simulink model "ADRC_Han"  (R2024b)
settings: Solver=VariableStepAuto  StartTime=0.0  StopTime=20  RelTol=1e-3
values from neighbouring files (symbols this model uses):
  A = [zeros(N, 1)  eye(N, N) ... (first row only)    [ADRC_Han_Vars.m]
  A_d_test = d_test_ss.A    [ADRC_Han_Vars.m]
  A_ESO_d = [1-l1_ESO_d, delta_t-l1_ESO_d*delta_t, 1/2 * delta_t^2 - 1/2 * l1_ESO_d*delta_t^2 ... (first row only)    [ADRC_Han_Vars.m]
  A_MESO_d = A_o_d - l_MESO_d*C_o_d*A_o_d    [ADRC_Han_Vars.m]
  A_o = [A_m e_m*c_T_d_m ... (first row only)    [ADRC_Han_Vars.m]
  A_O_d = A_m_d - l_o_d*C_m_d*A_m_d    [ADRC_Han_Vars.m]
  A_o_lqr = [A_m_lqr e_m*c_T_d_m_lqr ... (first row only)    [ADRC_Han_Vars.m]
  alpha_1 = 1    [ADRC_Han_Vars.m]
  alpha_2 = 1    [ADRC_Han_Vars.m]
  b = [zeros(N-1, 1) ... (first row only)    [ADRC_Han_Vars.m]
  b0 = K/T^2    (= 1.11111111111)    [ADRC_Han_Vars.m]
  B_d_test = d_test_ss.B    [ADRC_Han_Vars.m]
  b_ESO_d = [1/2*b0*delta_t^2 - l1_ESO_d*b0*delta_t^2 ... (first row only)    [ADRC_Han_Vars.m]
  B_MESO_d = B_o_d - l_MESO_d*C_o_d*B_o_d    [ADRC_Han_Vars.m]
  b_o = [b_m ... (first row only)    [ADRC_Han_Vars.m]
  B_O_d = B_m_d - l_o_d*C_m_d*B_m_d    [ADRC_Han_Vars.m]
  b_o_lqr = [b_m_lqr ... (first row only)    [ADRC_Han_Vars.m]
  beta_01 = 1    [ADRC_Han_Vars.m]
  beta_02 = 1 / (2*h^0.5)    (= 5)    [ADRC_Han_Vars.m]
  beta_03 = 2 / (5^2 * h^1.2)    (= 20.0950914521)    [ADRC_Han_Vars.m]
  c = 50    [ADRC_Han_Vars.m]
  C_d_test = d_test_ss.C    [ADRC_Han_Vars.m]
  c_o_T = [c_T_m 0]    [ADRC_Han_Vars.m]
  c_o_T_lqr = [c_T_m_lqr 0]    [ADRC_Han_Vars.m]
  c_t = [1, zeros(1, N)]    [ADRC_Han_Vars.m]
  D = 5    [ADRC_Han_Vars.m]
  delta = 0.05    [ADRC_Han_Vars.m]
  delta_t = 0.01    [ADRC_Han_Vars.m]
  h = 0.01    [ADRC_Han_Vars.m]
  h0 = 8*h    (= 0.08)    [ADRC_Han_Vars.m]
  K = 10    [ADRC_Han_Vars.m]
  k = ones(N,1)    [ADRC_Han_Vars.m]
  k1_c_d = (1 - z_cl)^2/delta_t^2    [ADRC_Han_Vars.m]
  k_c_T = acker(A_m,b_m, [-omega_cl,-omega_cl])    [ADRC_Han_Vars.m]
  k_c_T_dlqr = dlqr(A_m_dlqr,b_m_dlqr,Q,R)    [ADRC_Han_Vars.m]
  k_c_T_lqr = lqr(A_m_lqr,b_m_lqr,Q,R)    [ADRC_Han_Vars.m]
  k_d_T = (e_m*c_T_d_m) \ b_m    [ADRC_Han_Vars.m]
  k_d_T_lqr = (e_m*c_T_d_m_lqr) \ b_m_lqr    [ADRC_Han_Vars.m]
  k_dlqr = dlqr(A_m_d, B_m_d, Q, R)    [ADRC_Han_Vars.m]
  K_lqr = lqr(A_lqr,B_lqr,Q,R)    [ADRC_Han_Vars.m]
  k_o = acker(A_o',c_o_T',[-omega_O,-omega_O,-omega_O])'    [ADRC_Han_Vars.m]
  k_o_lqr = acker(A_o_lqr',c_o_T_lqr',[-omega_O,-omega_O,-omega_O])'    [ADRC_Han_Vars.m]
  k_s = -inv(c_T_m*inv(A_m-b_m*k_c_T)*b_m)    [ADRC_Han_Vars.m]
  k_s_dlqr = -inv(c_T_m*inv(A_m-b_m*k_dlqr)*b_m)    [ADRC_Han_Vars.m]
  k_s_lqr = -inv(c_T_m_lqr*inv(A_m_lqr-b_m_lqr*k_c_T_lqr)*b_m_lqr)    [ADRC_Han_Vars.m]
  K_s_lqr = -inv(C_lqr*inv(A_lqr-B_lqr*K_lqr)*B_lqr)    [ADRC_Han_Vars.m]
  k_T_d = [k1_c_d, k2_c_d]    [ADRC_Han_Vars.m]
  l = ones(N+1, 1)    [ADRC_Han_Vars.m]
  l_ESO_d = [l1_ESO_d, l2_ESO_d, l3_ESO_d]'    [ADRC_Han_Vars.m]
  l_MESO_d = acker(A_o_d',C_o_d',[z_MESO,z_MESO,z_MESO])'    [ADRC_Han_Vars.m]
  l_o_d = acker(A_m_d',C_m_d',[z_o,z_o])'    [ADRC_Han_Vars.m]
  N = 2    [ADRC_Han_Vars.m]
  r = 100000    [ADRC_Han_Vars.m]
  r0 = 2    [ADRC_Han_Vars.m]
  T = 3    [ADRC_Han_Vars.m]
undefined symbols (not defined in the file or in its folder): A_o_dlqr, b_o_dlqr, c_o_T_dlqr
libraries: simulink x2, slpidlib x1
settings Model: Creator=Henrik  LastModifiedBy=Henrik

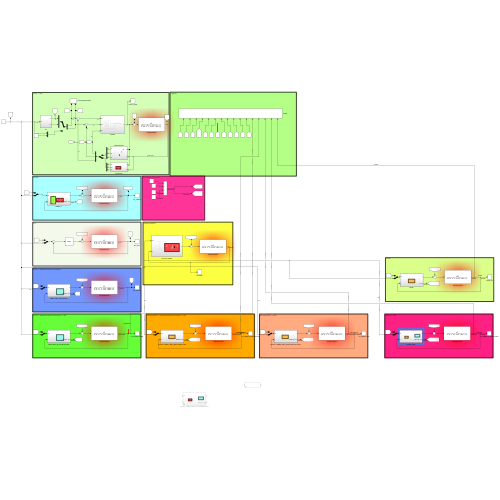
[thumbnail: Simulink's stored preview of the top-level diagram]
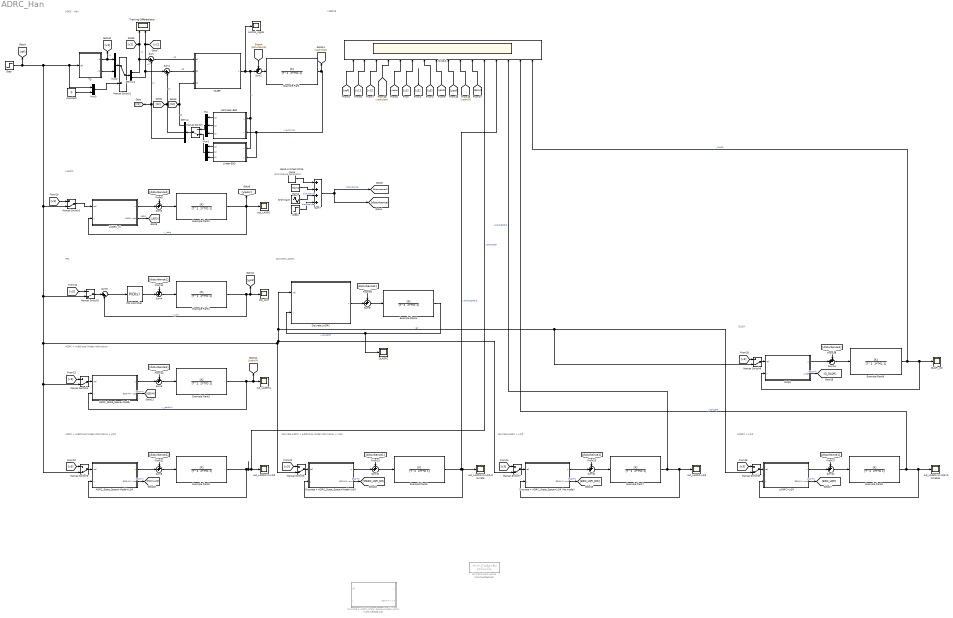
== system ADRC_Han ==
  note: Discrete LADRC
  note: Logging
  note: Disturbance Generation
  note: LADRC
  note: ADRC - Han
  note: PID
  note: ADRC + Additional Model Information
  note: ADRC + Additional Model Information + LQR
  note: Discrete ADRC + Additional Model Information + LQR
  note: Discrete ADRC + LQR
  note: LADRC + LQR
  note: DLQR
   Example Plant{,1..9} (10 alike) : TransferFcn  Numerator=[K]  Denominator="[T^2  2*T*D 1]"
  ADRC_State_Space+Model : Subsystem
  ADRC_State_Space+Model+LQR : Subsystem
  Band-Limited White Noise : simulink/Sources/Band-Limited White Noise  Cov=[0]  Ts=5  seed=[23341]
  Constant : Constant  Value=0
  DLADRC : Scope
  DLQR : Subsystem
  DLQR_out : Scope
  Demux : Demux  Outputs=3
  Demux1 : Demux  Outputs=2
  Discrete + ADRC_State_Space+LQR (No model) : Subsystem
  Discrete + ADRC_State_Space+Model+LQR : Subsystem
  Discrete + ADRC_State_Space+Model+LQR1 : Subsystem  Commented=on
  Discrete LADRC : Subsystem
  Discrete State-Space : DiscreteStateSpace  Commented=on  A=A_d_test  B=B_d_test  C=C_d_test  D=0  SampleTime=delta_t
  LADRC+LQR : Subsystem
  LADRC_ct : Subsystem
  Linear-ESO : Subsystem
  Manual Switch{,2..9} (9 alike) : ManualSwitch  CurrentSetting=0
  Manual Switch1 : ManualSwitch
  Mux : Mux  Inputs=3
  Mux1 : Mux  Inputs=3
  Mux2 : Mux  Inputs=2
  Mux3 : Mux  Inputs=2
  NLSEF : Subsystem
  Nonlinear-ESO : Subsystem
  Output : Scope  NumInputPorts=16
  PID Controller : slpidlib/PID Controller  Controller=PID  Form=Parallel  TimeDomain=Continuous-time  UseExternalTs=off  SampleTime=-1  IntegratorMethod=Forward Euler  FilterMethod=Forward Euler  ControllerParametersSource=internal  P=9.22990641554484  I=1.242622044959548  UseKiTs=off  D=-0.586776968571328  UseExternalDerivativeSource=off  N=0.165575426400758  UseFilter=on  TunerSelectOption=Transfer Function Based (PID Tuner App)  InitialConditionSource=internal  InitialConditionForIntegrator=0  InitialConditionForFilter=0  DifferentiatorICPrevScaledInput=0  ExternalReset=none  TrackingMode=off  Kt=1  LimitOutput=off  SatLimitsSource=internal  UpperSaturationLimit=inf  LowerSaturationLimit=-inf  LinearizeAsGain=on  AntiWindupMode=none  Kb=1  LimitIntegrator=off  UpperIntegratorSaturationLimit=inf  LowerIntegratorSaturationLimit=-inf  POutMin=[]  POutMax=[]  IOutMin=[]  IOutMax=[]  DOutMin=[]  DOutMax=[]  NOutMin=[]  NOutMax=[]  SumOutMin=[]  SumOutMax=[]  SaturationOutMin=[]  SaturationOutMax=[]  PParamMin=[]  PParamMax=[]  IParamMin=[]  IParamMax=[]  DParamMin=[]  DParamMax=[]  NParamMin=[]  NParamMax=[]  KbParamMin=[]  KbParamMax=[]  KtParamMin=[]  KtParamMax=[]  KbOutMin=[]  KbOutMax=[]  KtOutMin=[]  KtOutMax=[]  IntegratorOutMin=[]  IntegratorOutMax=[]  FilterOutMin=[]  FilterOutMax=[]  SumI1OutMin=[]  SumI1OutMax=[]  SumI2OutMin=[]  SumI2OutMax=[]  SumI3OutMin=[]  SumI3OutMax=[]  SumI4OutMin=[]  SumI4OutMax=[]  SumDOutMin=[]  SumDOutMax=[]  DifferentiatorOutMin=[]  DifferentiatorOutMax=[]  FilterDiffOutCoefMin=[]  FilterDiffOutCoefMax=[]  ReciprocalOutMin=[]  ReciprocalOutMax=[]  SumDenOutMin=[]  SumDenOutMax=[]  SumNumOutMin=[]  SumNumOutMax=[]  DivideOutMin=[]  DivideOutMax=[]  UdiffTsProdOutMin=[]  UdiffTsProdOutMax=[]  NTsProdOutMin=[]  NTsProdOutMax=[]  UintegralTsProdOutMin=[]  UintegralTsProdOutMax=[]  UngainTsProdOutMin=[]  UngainTsProdOutMax=[]  ClampingZeroOutDataTypeStr=Inherit: Inherit via back propagation  ClampingZeroOutMin=[]  ClampingZeroOutMax=[]  FilterDenConstantOutDataTypeStr=Inherit: Inherit via back propagation  FilterDenConstantOutMin=[]  FilterDenConstantOutMax=[]  PCopyOutDataTypeStr=Inherit: Inherit via back propagation  PCopyOutMin=[]  PCopyOutMax=[]  NCopyOutDataTypeStr=Inherit: Inherit via back propagation  NCopyOutMin=[]  NCopyOutMax=[]  IntegratorContinuousStateAttributes=''  IntegratorStateMustResolveToSignalObject=off  IntegratorRTWStateStorageClass=Auto  FilterContinuousStateAttributes=''  FilterStateMustResolveToSignalObject=off  FilterRTWStateStorageClass=Auto  ParallelPVariant=InternalParameters  IdealPVariant=Disabled  IVariant=InternalParameters  DVariant=InternalParameters  IntegratorVariant=Continuous  SatVariant=Disabled  AWVariant=Passthrough  PCopyVariant=Disabled  TRVariant=Disabled  FdbkBlocksVariant=Forward  IdealPFdbkVariant=Disabled  SatFdbkVariant=Disabled  DerivativeFilterVariant=ContFilter  NVariant=InternalParameters  NCopyVariant=Disabled  FilterICVariant=InternalICsFilter  IntegratorICVariant=InternalICs  ExternalResetVariant=Disabled  TRSumVariant=Passthrough  SumFdbkVariant=Disabled  SumVariant=Sum_PID  TsampFilterVariant=InternalTs  TsampNgainVariant=Passthrough  TsampIntegralVariant=Disabled_SignalSpec  ExternalSaturationOutDataTypeStr=Inherit: Same as second input  DerivativeSourceVariant=ErrorSignal  PreIntVariant=InternalPreInt
  PID_OUT : Scope
  Ramp : simulink/Sources/Ramp  slope=0  start=30  InitialOutput=0
  Sine Wave : Sin  Amplitude=0  Frequency=6  SampleTime=0
  Step : Step  SampleTime=0
  Step1 : Step  Time=10  After=0  SampleTime=0
  Sum : Sum  Inputs=|+-
  Sum1 : Sum  Inputs=|+-
  Sum{2..4,6,8..13} (10 alike) : Sum  Inputs=++|
  Sum5 : Sum  Inputs=|+-
  Sum7 : Sum  Inputs=++++
  TD : Subsystem
  Tracking Differentiator : Scope  NumInputPorts=2
  control_signal : Scope
  out_LADRC : Scope
  out_LADRC-LQR : Scope
  out_LADRC-M-LQR : Scope
  out_LADRC-M-LQR-Discrete : Scope
  out_LADRC-M-LQR-Discrete2 : Scope
  out_LADRC1 : Scope
  wires:
  NLSEF/1(u) -> control_signal/1, Sum2/2, Linear-ESO/1(u), Nonlinear-ESO/1(u)  "u"
  Demux1/1 -> Sum/1, [v1], Tracking Differentiator/1  "v1"
  Demux1/2 -> Tracking Differentiator/2, [v2], Sum1/1  "v2"
  Sum/1 -> NLSEF/1(e1)  "e1"
  Sum1/1 -> NLSEF/2(e2)  "e2"
  Demux/3 -> Sum/2, [z1]  "z1"
  Demux/2 -> Sum1/2, [z2]  "z2"
  Demux/1 -> NLSEF/3(z3), [z3]  "z3"
  " Example Plant"/1 -> Linear-ESO/2(y), Nonlinear-ESO/2(y), [yadrchan]  "y_adrc_han"
  [z1] -> Output/6
  [z2] -> ?
  [z3] -> Output/7
  Sum2/1 -> " Example Plant"/1
  [ref] -> Output/1
  " Example Plant2"/1 -> [yladrc], out_LADRC/1, LADRC_ct/2(y)  "y_ladrc"
  LADRC_ct/1(u) -> Sum3/2
  Sum3/1 -> " Example Plant2"/1
  [disturbance] -> Sum2/1
  [disturbance1] -> Sum3/1
  [yladrc] -> Output/5
  [v2] -> Output/3
  [v1] -> Output/2
  LADRC_ct/2(LESO - out) -> [LESO]  "LESO"
  [LESO] -> Output/8
  Nonlinear-ESO/2(z2) -> Mux/2
  Nonlinear-ESO/1(z3) -> Mux/1
  Nonlinear-ESO/3(z1) -> Mux/3
  Manual Switch/1 -> Demux/1
  Mux/1 -> Manual Switch/1
  Linear-ESO/2(z2) -> Mux1/2
  Linear-ESO/1(z3) -> Mux1/1
  Linear-ESO/3(z1) -> Mux1/3
  Mux1/1 -> Manual Switch/2
  TD/2(v2) -> Mux2/2
  TD/1(v1) -> Mux2/1, [v3]  "v1"
  Mux2/1 -> Manual Switch1/1
  Manual Switch1/1 -> Demux1/1
  Mux3/1 -> Manual Switch1/2
  Constant/1 -> Mux3/2
  [v3] -> Manual Switch2/1
  Manual Switch2/1 -> LADRC_ct/1(ref)
  " Example Plant1"/1 -> Sum5/2, [ypid], PID_OUT/1  "y_pid"
  Sum4/1 -> " Example Plant1"/1
  [disturbance1] -> Sum4/1
  PID Controller/1 -> Sum4/2
  [v3] -> Manual Switch3/1
  Manual Switch3/1 -> Sum5/1
  Sum5/1 -> PID Controller/1
  " Example Plant3"/1 -> out_LADRC1/1, [yadrcM], ADRC_State_Space+Model/2(y)  "y_adrc+M"
  Manual Switch4/1 -> ADRC_State_Space+Model/1(ref)
  Sum6/1 -> " Example Plant3"/1
  [v3] -> Manual Switch4/1
  [disturbance1] -> Sum6/1
  ADRC_State_Space+Model/1(u) -> Sum6/2
  Sum7/1 -> [disturbance], [disturbance1]  "disturbance"
  [ypid] -> Output/9
  [yadrcM] -> Output/10
  ADRC_State_Space+Model/2(ESO+M - out) -> [ESOM]  "ESO+M"
  [ESOM] -> Output/11
  [yadrchan] -> Output/4
  Step1/1 -> Sum7/4  "disturbance"
  Sine Wave/1 -> Sum7/3  "disturbance"
  Ramp/1 -> Sum7/2
  Band-Limited White Noise/1 -> Sum7/1
  " Example Plant4"/1 -> DLADRC/1, Discrete LADRC/2(y)  "y_DLADRC"
  Discrete LADRC/1(u) -> Sum8/2
  [disturbance1] -> Sum8/1
  Sum8/1 -> " Example Plant4"/1
  Sum9/1 -> " Example Plant5"/1
  [v3] -> Manual Switch5/1
  ADRC_State_Space+Model+LQR/2(ESO+M - out) -> [ESOM_LQR]  "ESO+M"
  ADRC_State_Space+Model+LQR/1(u) -> Sum9/2
  " Example Plant5"/1 -> Output/12, out_LADRC-M-LQR/1, ADRC_State_Space+Model+LQR/2(y)  "yadrcMLQR"
  [disturbance1] -> Sum9/1
  Manual Switch5/1 -> ADRC_State_Space+Model+LQR/1(ref)
  Manual Switch6/1 -> Discrete + ADRC_State_Space+Model+LQR/1(ref)
  Discrete + ADRC_State_Space+Model+LQR/1(u) -> Sum10/2
  " Example Plant6"/1 -> Output/13, out_LADRC-M-LQR-Discrete/1, Discrete + ADRC_State_Space+Model+LQR/2(y)  "yadrcMLQRDIS"
  Discrete + ADRC_State_Space+Model+LQR/2(ESO+M - out) -> [MESO_LQR_DIS]  "ESO+M"
  [disturbance1] -> Sum10/1
  Sum10/1 -> " Example Plant6"/1
  [v3] -> Manual Switch6/1
  Sum11/1 -> " Example Plant7"/1
  [v3] -> Manual Switch7/1
  Discrete + ADRC_State_Space+LQR (No model)/1(u) -> Sum11/2
  Manual Switch7/1 -> Discrete + ADRC_State_Space+LQR (No model)/1(ref)
  " Example Plant7"/1 -> out_LADRC-LQR/1, Discrete + ADRC_State_Space+LQR (No model)/2(y), Output/14  "yadrcLQRDIS"
  [disturbance1] -> Sum11/1
  Discrete + ADRC_State_Space+LQR (No model)/2(ESO+M - out) -> [ESO_LQR_DIS]  "ESO+M"
  LADRC+LQR/2(ESO+M - out) -> [ESO_LQR]  "ESO+M"
  " Example Plant8"/1 -> Output/15, out_LADRC-M-LQR-Discrete2/1, LADRC+LQR/2(y)  "yadrcLQR"
  [disturbance1] -> Sum12/1
  LADRC+LQR/1(u) -> Sum12/2
  Manual Switch8/1 -> LADRC+LQR/1(ref)
  [v3] -> Manual Switch8/1
  Sum12/1 -> " Example Plant8"/1
  Step/1 -> Mux3/1, TD/1(ref), Manual Switch5/2, Manual Switch4/2, Manual Switch6/2, Manual Switch7/2, Discrete LADRC/1(ref), Manual Switch9/2, Manual Switch8/2, Manual Switch3/2, Manual Switch2/2, [ref]  "ref"
  Manual Switch9/1 -> DLQR/1(ref)
  DLQR/2(x_hat) -> [O_DLQR]  "ESO+M"
  Sum13/1 -> " Example Plant9"/1
  [v3] -> Manual Switch9/1
  DLQR/1(u) -> Sum13/2
  " Example Plant9"/1 -> DLQR_out/1, DLQR/2(y), Output/16  "yDLQR"
  [disturbance1] -> Sum13/1

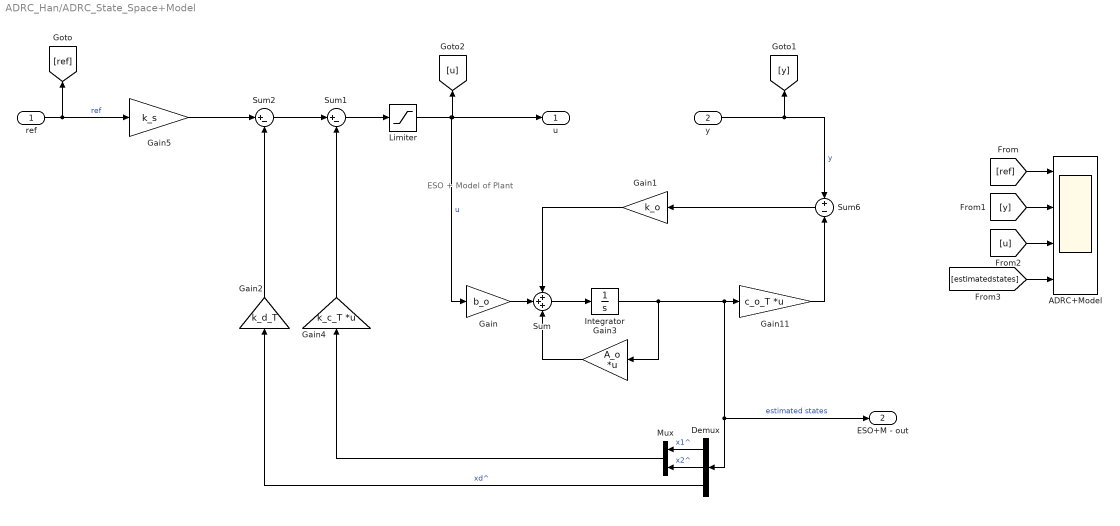
== system ADRC_Han/ADRC_State_Space+Model ==
  note: ESO + Model of Plant
  ref : Inport
  y : Inport  Port=2
  ADRC+Model : Scope  NumInputPorts=4
  Demux : Demux  Outputs=N+1
  Gain : Gain  Gain=b_o
  Gain1 : Gain  Gain=k_o
  Gain11 : Gain  Gain=c_o_T  Multiplication=Matrix(K*u)
  Gain2 : Gain  Gain=k_d_T
  Gain3 : Gain  Gain=A_o  Multiplication=Matrix(K*u)
  Gain4 : Gain  Gain=k_c_T  Multiplication=Matrix(K*u)
  Gain5 : Gain  Gain=k_s
  Integrator : Integrator
  Limiter : Saturate  UpperLimit=r  LowerLimit=-r
  Mux : Mux  Inputs=2
  Sum : Sum  Inputs=+++
  Sum1 : Sum  Inputs=|+-
  Sum2 : Sum  Inputs=|+-
  Sum6 : Sum  Inputs=+|-
  u : Outport
  ESO+M - out : Outport  Port=2
  wires:
  Limiter/1 -> [u], u/1, Gain/1  "u"
  Integrator/1 -> Gain3/1, ESO+M - out/1, Demux/1, Gain11/1  "estimated states"
  Gain11/1 -> Sum6/2
  ref/1 -> Gain5/1, [ref]  "ref"
  y/1 -> Sum6/1, [y]  "y"
  [ref] -> ADRC+Model/1
  [y] -> ADRC+Model/2
  [u] -> ADRC+Model/3
  [estimatedstates] -> ADRC+Model/4
  Sum6/1 -> Gain1/1
  Gain/1 -> Sum/2
  Gain1/1 -> Sum/1
  Sum/1 -> Integrator/1
  Gain3/1 -> Sum/3
  Demux/1 -> Mux/1  "x1^"
  Demux/2 -> Mux/2  "x2^"
  Demux/3 -> Gain2/1  "xd^"
  Sum1/1 -> Limiter/1
  Mux/1 -> Gain4/1
  Gain4/1 -> Sum1/2
  Gain2/1 -> Sum2/2
  Sum2/1 -> Sum1/1
  Gain5/1 -> Sum2/1

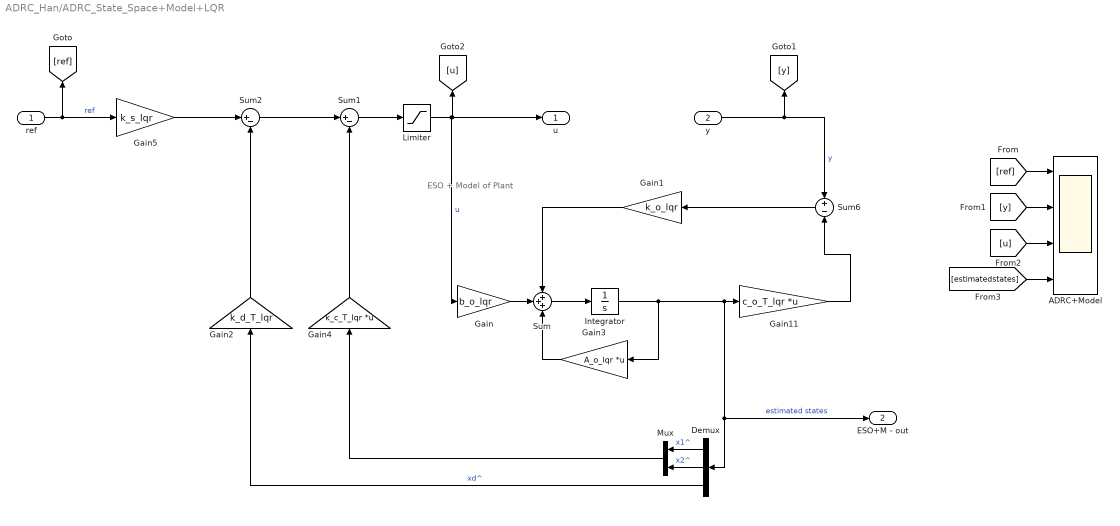
== system ADRC_Han/ADRC_State_Space+Model+LQR ==
  note: ESO + Model of Plant
  ref : Inport
  y : Inport  Port=2
  ADRC+Model : Scope  NumInputPorts=4
  Demux : Demux  Outputs=N+1
  Gain : Gain  Gain=b_o_lqr
  Gain1 : Gain  Gain=k_o_lqr
  Gain11 : Gain  Gain=c_o_T_lqr  Multiplication=Matrix(K*u)
  Gain2 : Gain  Gain=k_d_T_lqr
  Gain3 : Gain  Gain=A_o_lqr  Multiplication=Matrix(K*u)
  Gain4 : Gain  Gain=k_c_T_lqr  Multiplication=Matrix(K*u)
  Gain5 : Gain  Gain=k_s_lqr
  Integrator : Integrator
  Limiter : Saturate  UpperLimit=r  LowerLimit=-r
  Mux : Mux  Inputs=2
  Sum : Sum  Inputs=+++
  Sum1 : Sum  Inputs=|+-
  Sum2 : Sum  Inputs=|+-
  Sum6 : Sum  Inputs=+|-
  u : Outport
  ESO+M - out : Outport  Port=2
  wires:
  Limiter/1 -> [u], u/1, Gain/1  "u"
  Integrator/1 -> Gain3/1, ESO+M - out/1, Demux/1, Gain11/1  "estimated states"
  Gain11/1 -> Sum6/2
  ref/1 -> Gain5/1, [ref]  "ref"
  y/1 -> Sum6/1, [y]  "y"
  [ref] -> ADRC+Model/1
  [y] -> ADRC+Model/2
  [u] -> ADRC+Model/3
  [estimatedstates] -> ADRC+Model/4
  Sum6/1 -> Gain1/1
  Gain/1 -> Sum/2
  Gain1/1 -> Sum/1
  Sum/1 -> Integrator/1
  Gain3/1 -> Sum/3
  Demux/1 -> Mux/1  "x1^"
  Demux/2 -> Mux/2  "x2^"
  Demux/3 -> Gain2/1  "xd^"
  Sum1/1 -> Limiter/1
  Mux/1 -> Gain4/1
  Gain4/1 -> Sum1/2
  Gain2/1 -> Sum2/2
  Sum2/1 -> Sum1/1
  Gain5/1 -> Sum2/1

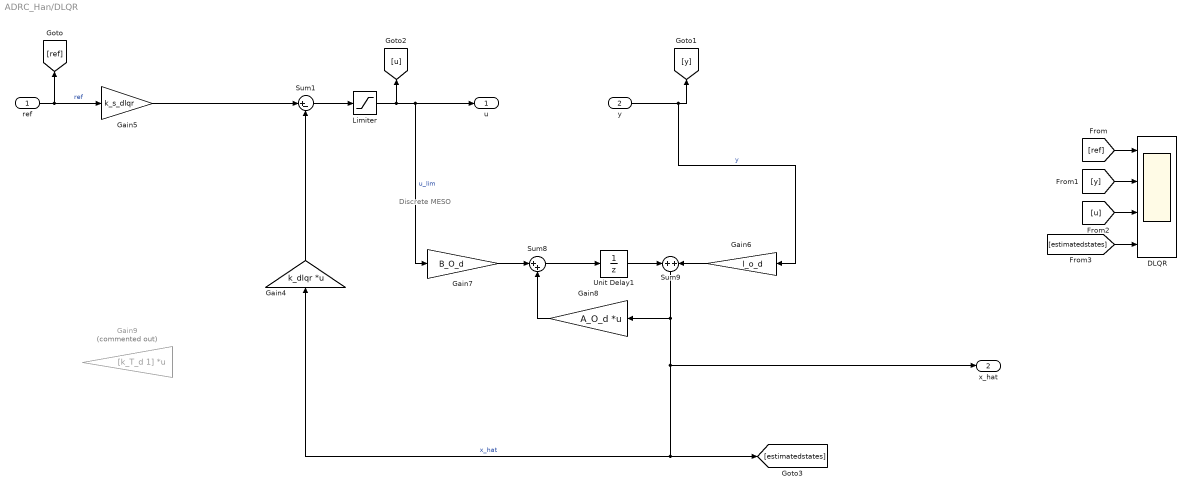
== system ADRC_Han/DLQR ==
  note: Discrete MESO
  ref : Inport
  y : Inport  Port=2
  DLQR : Scope  NumInputPorts=4
  Gain4 : Gain  Gain=k_dlqr  Multiplication=Matrix(K*u)
  Gain5 : Gain  Gain=k_s_dlqr
  Gain6 : Gain  Gain=l_o_d
  Gain7 : Gain  Gain=B_O_d
  Gain8 : Gain  Gain=A_O_d  Multiplication=Matrix(K*u)
  Gain9 : Gain  Commented=on  Gain=[k_T_d 1]  Multiplication=Matrix(K*u)
  Limiter : Saturate  UpperLimit=r  LowerLimit=-r
  Sum1 : Sum  Inputs=|+-
  Sum8 : Sum  Inputs=|++
  Sum9 : Sum  Inputs=+|+
  Unit Delay1 : UnitDelay  SampleTime=delta_t  HasFrameUpgradeWarning=on
  u : Outport
  x_hat : Outport  Port=2
  wires:
  ref/1 -> Gain5/1, [ref]  "ref"
  [ref] -> DLQR/1
  [y] -> DLQR/2
  [u] -> DLQR/3
  [estimatedstates] -> DLQR/4
  Sum1/1 -> Limiter/1
  Gain4/1 -> Sum1/2
  Gain5/1 -> Sum1/1
  Limiter/1 -> Gain7/1, u/1, [u]  "u_lim"
  Sum9/1 -> Gain4/1, [estimatedstates], x_hat/1, Gain8/1  "x_hat"
  Gain6/1 -> Sum9/2
  Sum8/1 -> Unit Delay1/1
  y/1 -> Gain6/1, [y]  "y"
  Unit Delay1/1 -> Sum9/1
  Gain7/1 -> Sum8/1
  Gain8/1 -> Sum8/2

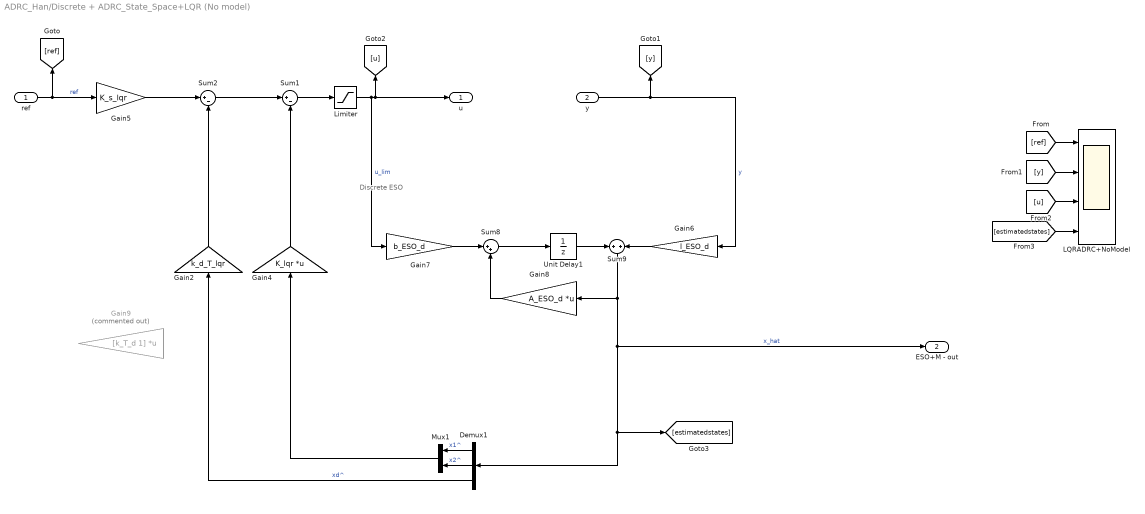
== system ADRC_Han/Discrete + ADRC_State_Space+LQR (No model) ==
  note: Discrete ESO
  ref : Inport
  y : Inport  Port=2
  Demux1 : Demux  Outputs=N+1
  Gain2 : Gain  Gain=k_d_T_lqr
  Gain4 : Gain  Gain=K_lqr  Multiplication=Matrix(K*u)
  Gain5 : Gain  Gain=K_s_lqr
  Gain6 : Gain  Gain=l_ESO_d
  Gain7 : Gain  Gain=b_ESO_d
  Gain8 : Gain  Gain=A_ESO_d  Multiplication=Matrix(K*u)
  Gain9 : Gain  Commented=on  Gain=[k_T_d 1]  Multiplication=Matrix(K*u)
  LQRADRC+NoModel : Scope  NumInputPorts=4
  Limiter : Saturate  UpperLimit=r  LowerLimit=-r
  Mux1 : Mux  Inputs=2
  Sum1 : Sum  Inputs=|+-
  Sum2 : Sum  Inputs=|+-
  Sum8 : Sum  Inputs=|++
  Sum9 : Sum  Inputs=+|+
  Unit Delay1 : UnitDelay  SampleTime=delta_t  HasFrameUpgradeWarning=on
  u : Outport
  ESO+M - out : Outport  Port=2
  wires:
  ref/1 -> Gain5/1, [ref]  "ref"
  y/1 -> Gain6/1, [y]  "y"
  [ref] -> LQRADRC+NoModel/1
  [y] -> LQRADRC+NoModel/2
  [u] -> LQRADRC+NoModel/3
  [estimatedstates] -> LQRADRC+NoModel/4
  Sum1/1 -> Limiter/1
  Gain4/1 -> Sum1/2
  Gain2/1 -> Sum2/2
  Sum2/1 -> Sum1/1
  Gain5/1 -> Sum2/1
  Sum8/1 -> Unit Delay1/1
  Gain8/1 -> Sum8/2
  Unit Delay1/1 -> Sum9/1
  Gain7/1 -> Sum8/1
  Limiter/1 -> u/1, [u], Gain7/1  "u_lim"
  Sum9/1 -> Demux1/1, [estimatedstates], ESO+M - out/1, Gain8/1  "x_hat"
  Gain6/1 -> Sum9/2
  Demux1/1 -> Mux1/1  "x1^"
  Mux1/1 -> Gain4/1
  Demux1/2 -> Mux1/2  "x2^"
  Demux1/3 -> Gain2/1  "xd^"

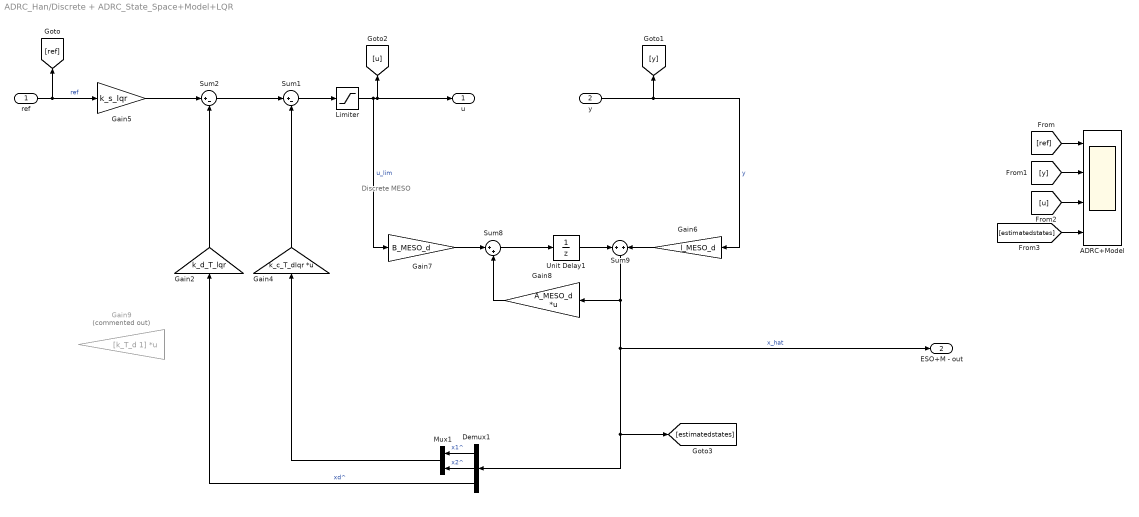
== system ADRC_Han/Discrete + ADRC_State_Space+Model+LQR ==
  note: Discrete MESO
  ref : Inport
  y : Inport  Port=2
  ADRC+Model : Scope  NumInputPorts=4
  Demux1 : Demux  Outputs=N+1
  Gain2 : Gain  Gain=k_d_T_lqr
  Gain4 : Gain  Gain=k_c_T_dlqr  Multiplication=Matrix(K*u)
  Gain5 : Gain  Gain=k_s_lqr
  Gain6 : Gain  Gain=l_MESO_d
  Gain7 : Gain  Gain=B_MESO_d
  Gain8 : Gain  Gain=A_MESO_d  Multiplication=Matrix(K*u)
  Gain9 : Gain  Commented=on  Gain=[k_T_d 1]  Multiplication=Matrix(K*u)
  Limiter : Saturate  UpperLimit=r  LowerLimit=-r
  Mux1 : Mux  Inputs=2
  Sum1 : Sum  Inputs=|+-
  Sum2 : Sum  Inputs=|+-
  Sum8 : Sum  Inputs=|++
  Sum9 : Sum  Inputs=+|+
  Unit Delay1 : UnitDelay  SampleTime=delta_t  HasFrameUpgradeWarning=on
  u : Outport
  ESO+M - out : Outport  Port=2
  wires:
  ref/1 -> Gain5/1, [ref]  "ref"
  y/1 -> Gain6/1, [y]  "y"
  [ref] -> ADRC+Model/1
  [y] -> ADRC+Model/2
  [u] -> ADRC+Model/3
  [estimatedstates] -> ADRC+Model/4
  Sum1/1 -> Limiter/1
  Gain4/1 -> Sum1/2
  Gain2/1 -> Sum2/2
  Sum2/1 -> Sum1/1
  Gain5/1 -> Sum2/1
  Sum8/1 -> Unit Delay1/1
  Gain8/1 -> Sum8/2
  Unit Delay1/1 -> Sum9/1
  Gain7/1 -> Sum8/1
  Limiter/1 -> u/1, [u], Gain7/1  "u_lim"
  Sum9/1 -> Demux1/1, [estimatedstates], ESO+M - out/1, Gain8/1  "x_hat"
  Gain6/1 -> Sum9/2
  Demux1/1 -> Mux1/1  "x1^"
  Mux1/1 -> Gain4/1
  Demux1/2 -> Mux1/2  "x2^"
  Demux1/3 -> Gain2/1  "xd^"

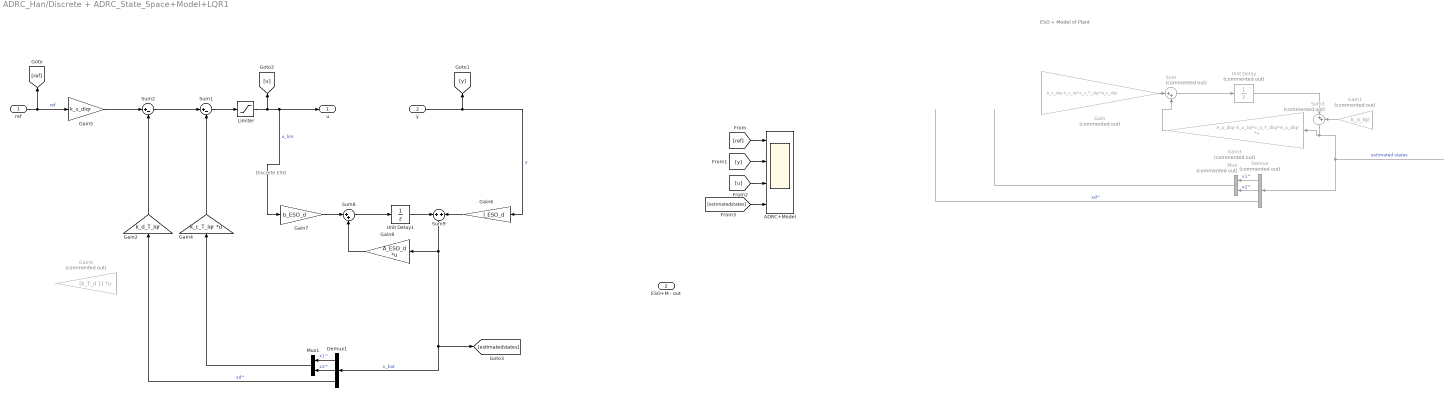
== system ADRC_Han/Discrete + ADRC_State_Space+Model+LQR1 ==
  note: Discrete ESO
  note: ESO + Model of Plant
  ref : Inport
  y : Inport  Port=2
  ADRC+Model : Scope  NumInputPorts=4
  Demux : Demux  Commented=on  Outputs=N+1
  Demux1 : Demux  Outputs=N+1
  Gain : Gain  Commented=on  Gain=b_o_dlqr-k_o_lqr*c_o_T_dlqr*b_o_dlqr
  Gain1 : Gain  Commented=on  Gain=k_o_lqr
  Gain2 : Gain  Gain=k_d_T_lqr
  Gain3 : Gain  Commented=on  Gain=A_o_dlqr-k_o_lqr*c_o_T_dlqr*A_o_dlqr  Multiplication=Matrix(K*u)
  Gain4 : Gain  Gain=k_c_T_lqr  Multiplication=Matrix(K*u)
  Gain5 : Gain  Gain=k_s_dlqr
  Gain6 : Gain  Gain=l_ESO_d
  Gain7 : Gain  Gain=b_ESO_d
  Gain8 : Gain  Gain=A_ESO_d  Multiplication=Matrix(K*u)
  Gain9 : Gain  Commented=on  Gain=[k_T_d 1]  Multiplication=Matrix(K*u)
  Limiter : Saturate  UpperLimit=r  LowerLimit=-r
  Mux : Mux  Commented=on  Inputs=2
  Mux1 : Mux  Inputs=2
  Sum : Sum  Commented=on  Inputs=|++
  Sum1 : Sum  Inputs=|+-
  Sum2 : Sum  Inputs=|+-
  Sum3 : Sum  Commented=on  Inputs=|++
  Sum8 : Sum  Inputs=|++
  Sum9 : Sum  Inputs=+|+
  Unit Delay : UnitDelay  Commented=on  SampleTime=delta_t  HasFrameUpgradeWarning=on
  Unit Delay1 : UnitDelay  SampleTime=delta_t  HasFrameUpgradeWarning=on
  u : Outport
  ESO+M - out : Outport  Port=2
  wires:
  ref/1 -> Gain5/1, [ref]  "ref"
  y/1 -> Gain6/1, [y]  "y"
  [ref] -> ADRC+Model/1
  [y] -> ADRC+Model/2
  [u] -> ADRC+Model/3
  [estimatedstates] -> ADRC+Model/4
  Sum1/1 -> Limiter/1
  Gain4/1 -> Sum1/2
  Gain2/1 -> Sum2/2
  Sum2/1 -> Sum1/1
  Gain5/1 -> Sum2/1
  Sum8/1 -> Unit Delay1/1
  Gain8/1 -> Sum8/2
  Unit Delay1/1 -> Sum9/1
  Gain7/1 -> Sum8/1
  Limiter/1 -> [u], Gain7/1, u/1  "u_lim"
  Sum9/1 -> Demux1/1, [estimatedstates], Gain8/1  "x_hat"
  Gain6/1 -> Sum9/2
  Demux/3 -> ?  "xd^"
  Sum/1 -> Unit Delay/1
  Demux/2 -> Mux/2  "x2^"
  ? -> Gain/1  "u"
  Demux/1 -> Mux/1  "x1^"
  Sum3/1 -> Gain3/1, Demux/1  "estimated states"
  ? -> Gain1/1  "y"
  Mux/1 -> ?
  Unit Delay/1 -> Sum3/1
  Gain3/1 -> Sum/2
  Gain/1 -> Sum/1
  Gain1/1 -> Sum3/2
  Demux1/1 -> Mux1/1  "x1^"
  Mux1/1 -> Gain4/1
  Demux1/2 -> Mux1/2  "x2^"
  Demux1/3 -> Gain2/1  "xd^"

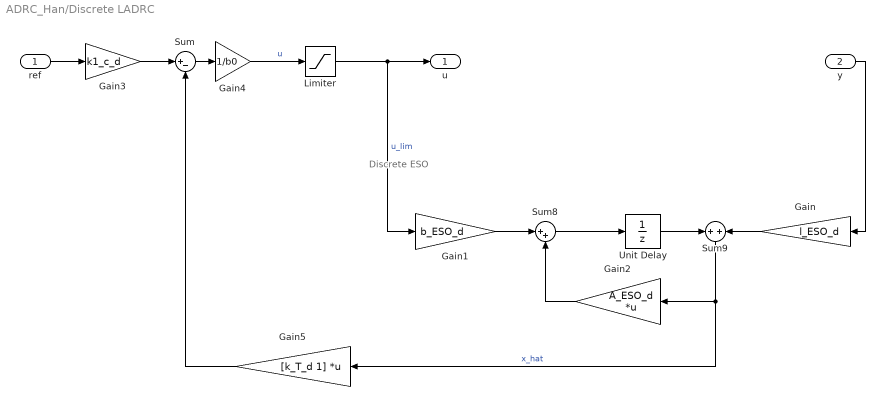
== system ADRC_Han/Discrete LADRC ==
  note: Discrete ESO
  ref : Inport
  y : Inport  Port=2
  Gain : Gain  Gain=l_ESO_d
  Gain1 : Gain  Gain=b_ESO_d
  Gain2 : Gain  Gain=A_ESO_d  Multiplication=Matrix(K*u)
  Gain3 : Gain  Gain=k1_c_d
  Gain4 : Gain  Gain=1/b0
  Gain5 : Gain  Gain=[k_T_d 1]  Multiplication=Matrix(K*u)
  Limiter : Saturate  UpperLimit=r  LowerLimit=-r
  Sum : Sum  Inputs=|+-
  Sum8 : Sum  Inputs=|++
  Sum9 : Sum  Inputs=+|+
  Unit Delay : UnitDelay  SampleTime=delta_t  HasFrameUpgradeWarning=on
  u : Outport
  wires:
  Gain1/1 -> Sum8/1
  Unit Delay/1 -> Sum9/1
  Sum8/1 -> Unit Delay/1
  Sum9/1 -> Gain5/1, Gain2/1  "x_hat"
  Gain/1 -> Sum9/2
  Gain2/1 -> Sum8/2
  Gain4/1 -> Limiter/1  "u"
  ref/1 -> Gain3/1
  Gain3/1 -> Sum/1
  Sum/1 -> Gain4/1
  Limiter/1 -> Gain1/1, u/1  "u_lim"
  y/1 -> Gain/1
  Gain5/1 -> Sum/2

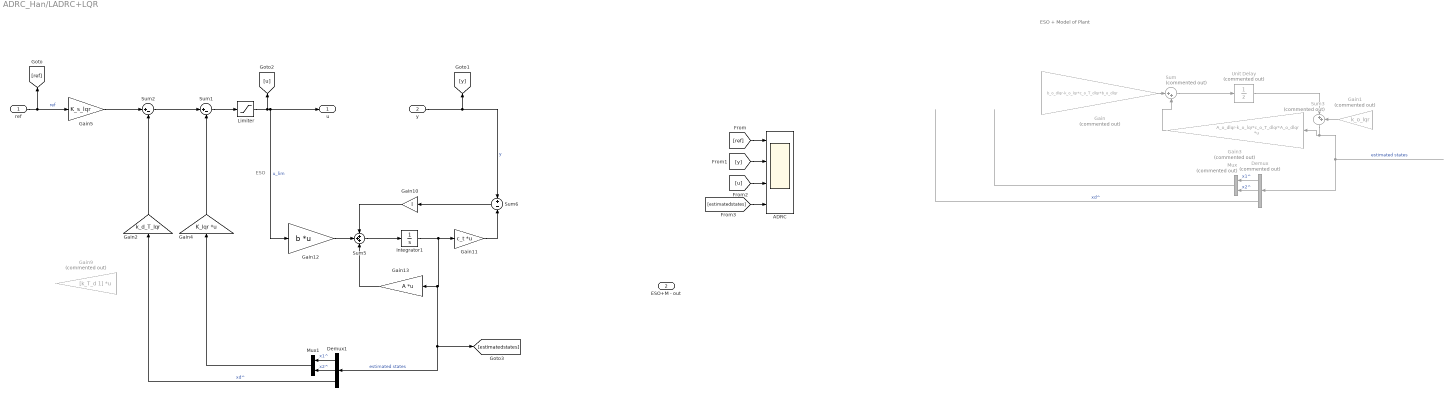
== system ADRC_Han/LADRC+LQR ==
  note: ESO
  note: ESO + Model of Plant
  ref : Inport
  y : Inport  Port=2
  ADRC : Scope  NumInputPorts=4
  Demux : Demux  Commented=on  Outputs=N+1
  Demux1 : Demux  Outputs=N+1
  Gain : Gain  Commented=on  Gain=b_o_dlqr-k_o_lqr*c_o_T_dlqr*b_o_dlqr
  Gain1 : Gain  Commented=on  Gain=k_o_lqr
  Gain10 : Gain  Gain=l
  Gain11 : Gain  Gain=c_t  Multiplication=Matrix(K*u)
  Gain12 : Gain  Gain=b  Multiplication=Matrix(K*u)
  Gain13 : Gain  Gain=A  Multiplication=Matrix(K*u)
  Gain2 : Gain  Gain=k_d_T_lqr
  Gain3 : Gain  Commented=on  Gain=A_o_dlqr-k_o_lqr*c_o_T_dlqr*A_o_dlqr  Multiplication=Matrix(K*u)
  Gain4 : Gain  Gain=K_lqr  Multiplication=Matrix(K*u)
  Gain5 : Gain  Gain=K_s_lqr
  Gain9 : Gain  Commented=on  Gain=[k_T_d 1]  Multiplication=Matrix(K*u)
  Integrator1 : Integrator
  Limiter : Saturate  UpperLimit=r  LowerLimit=-r
  Mux : Mux  Commented=on  Inputs=2
  Mux1 : Mux  Inputs=2
  Sum : Sum  Commented=on  Inputs=|++
  Sum1 : Sum  Inputs=|+-
  Sum2 : Sum  Inputs=|+-
  Sum3 : Sum  Commented=on  Inputs=|++
  Sum5 : Sum  Inputs=+++
  Sum6 : Sum  Inputs=+|-
  Unit Delay : UnitDelay  Commented=on  SampleTime=delta_t  HasFrameUpgradeWarning=on
  u : Outport
  ESO+M - out : Outport  Port=2
  wires:
  ref/1 -> Gain5/1, [ref]  "ref"
  y/1 -> Sum6/1, [y]  "y"
  [ref] -> ADRC/1
  [y] -> ADRC/2
  [u] -> ADRC/3
  [estimatedstates] -> ADRC/4
  Sum1/1 -> Limiter/1
  Gain4/1 -> Sum1/2
  Gain2/1 -> Sum2/2
  Sum2/1 -> Sum1/1
  Gain5/1 -> Sum2/1
  Demux/3 -> ?  "xd^"
  Sum/1 -> Unit Delay/1
  Demux/2 -> Mux/2  "x2^"
  ? -> Gain/1  "u"
  Demux/1 -> Mux/1  "x1^"
  Sum3/1 -> Gain3/1, Demux/1  "estimated states"
  ? -> Gain1/1  "y"
  Mux/1 -> ?
  Unit Delay/1 -> Sum3/1
  Gain3/1 -> Sum/2
  Gain/1 -> Sum/1
  Gain1/1 -> Sum3/2
  Demux1/1 -> Mux1/1  "x1^"
  Mux1/1 -> Gain4/1
  Demux1/2 -> Mux1/2  "x2^"
  Demux1/3 -> Gain2/1  "xd^"
  Gain11/1 -> Sum6/2
  Gain12/1 -> Sum5/2
  Limiter/1 -> Gain12/1, u/1, [u]  "u_lim"
  Integrator1/1 -> Gain11/1, Demux1/1, [estimatedstates], Gain13/1  "estimated states"
  Gain10/1 -> Sum5/1
  Sum5/1 -> Integrator1/1
  Sum6/1 -> Gain10/1
  Gain13/1 -> Sum5/3

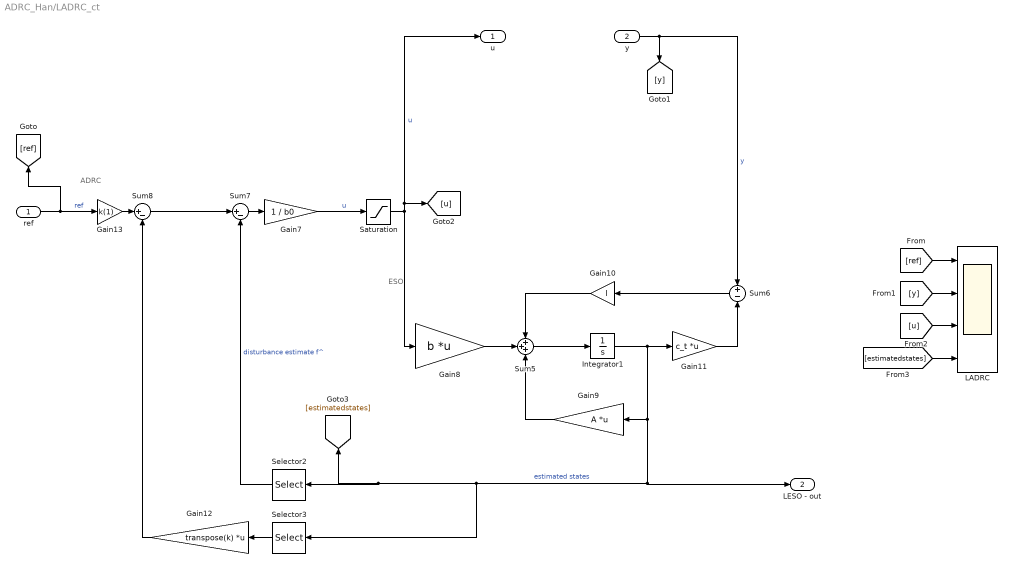
== system ADRC_Han/LADRC_ct ==
  note: ESO
  note: ADRC
  ref : Inport
  y : Inport  Port=2
  Gain10 : Gain  Gain=l
  Gain11 : Gain  Gain=c_t  Multiplication=Matrix(K*u)
  Gain12 : Gain  Gain=transpose(k)  Multiplication=Matrix(K*u)
  Gain13 : Gain  Gain=k(1)
  Gain7 : Gain  Gain=1 / b0
  Gain8 : Gain  Gain=b  Multiplication=Matrix(K*u)
  Gain9 : Gain  Gain=A  Multiplication=Matrix(K*u)
  Integrator1 : Integrator
  LADRC : Scope  NumInputPorts=4
  Saturation : Saturate  UpperLimit=r  LowerLimit=-r
  Selector2 : Selector  InputPortWidth=N+1  IndexOptions=Index vector (dialog)  Indices=[N+1]  OutputSizes=1
  Selector3 : Selector  InputPortWidth=N+1  IndexOptions=Index vector (dialog)  Indices=[1:N]  OutputSizes=1
  Sum5 : Sum  Inputs=+++
  Sum6 : Sum  Inputs=+|-
  Sum7 : Sum  Inputs=|+-
  Sum8 : Sum  Inputs=|+-
  u : Outport
  LESO - out : Outport  Port=2
  wires:
  Gain8/1 -> Sum5/2
  Saturation/1 -> [u], u/1, Gain8/1  "u"
  Integrator1/1 -> Gain11/1, LESO - out/1, Selector3/1, [estimatedstates], Selector2/1, Gain9/1  "estimated states"
  Gain11/1 -> Sum6/2
  Sum6/1 -> Gain10/1
  Selector2/1 -> Sum7/2  "disturbance estimate f^"
  Sum7/1 -> Gain7/1
  Gain12/1 -> Sum8/2
  Gain10/1 -> Sum5/1
  Gain9/1 -> Sum5/3
  Gain13/1 -> Sum8/1
  Sum5/1 -> Integrator1/1
  Selector3/1 -> Gain12/1
  Sum8/1 -> Sum7/1
  ref/1 -> Gain13/1, [ref]  "ref"
  y/1 -> Sum6/1, [y]  "y"
  [ref] -> LADRC/1
  [y] -> LADRC/2
  [u] -> LADRC/3
  [estimatedstates] -> LADRC/4
  Gain7/1 -> Saturation/1  "u"

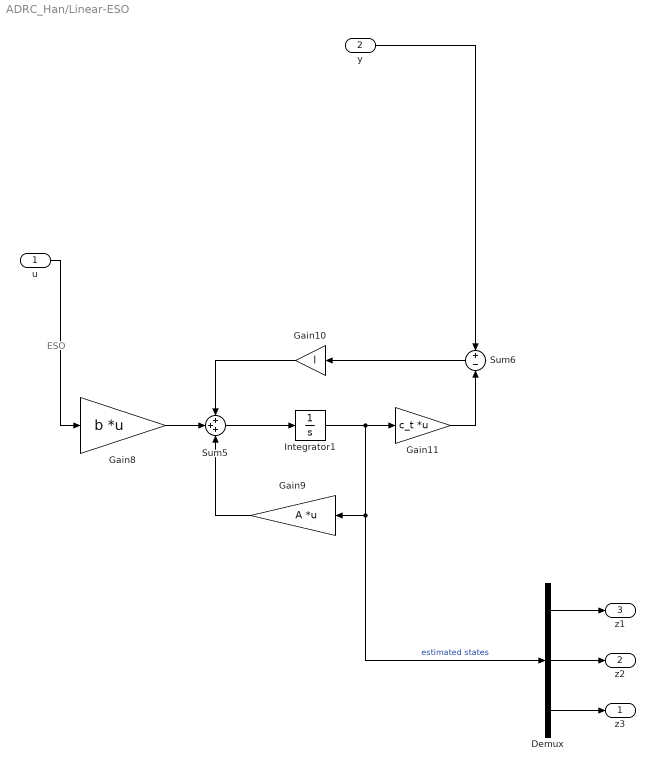
== system ADRC_Han/Linear-ESO ==
  note: ESO
  u : Inport
  y : Inport  Port=2
  Demux : Demux  Outputs=3
  Gain10 : Gain  Gain=l
  Gain11 : Gain  Gain=c_t  Multiplication=Matrix(K*u)
  Gain8 : Gain  Gain=b  Multiplication=Matrix(K*u)
  Gain9 : Gain  Gain=A  Multiplication=Matrix(K*u)
  Integrator1 : Integrator
  Sum5 : Sum  Inputs=+++
  Sum6 : Sum  Inputs=+|-
  z3 : Outport
  z2 : Outport  Port=2
  z1 : Outport  Port=3
  wires:
  Gain10/1 -> Sum5/1
  Integrator1/1 -> Gain11/1, Demux/1, Gain9/1  "estimated states"
  Gain8/1 -> Sum5/2
  Gain11/1 -> Sum6/2
  y/1 -> Sum6/1
  Sum6/1 -> Gain10/1
  Gain9/1 -> Sum5/3
  Sum5/1 -> Integrator1/1
  u/1 -> Gain8/1
  Demux/1 -> z1/1
  Demux/2 -> z2/1
  Demux/3 -> z3/1

== system ADRC_Han/NLSEF ==
  e1 : Inport
  e2 : Inport  Port=2
  z3 : Inport  Port=3
  Constant : Constant  Value=r
  Constant1 : Constant  Value=h
  Gain : Gain  Gain=c
  Gain1 : Gain  Gain=b0
  Gain2 : Gain  Gain=-1
  MATLAB Function : MATLAB Function  TreatAsAtomicUnit=on  SystemSampleTime=h
  Sum : Sum  Inputs=|++
  u : Outport
  wires:
  e1/1 -> MATLAB Function/1(e1)
  Gain/1 -> MATLAB Function/2(e2)
  e2/1 -> Gain/1
  Constant1/1 -> MATLAB Function/4(h)
  Constant/1 -> MATLAB Function/3(r)
  MATLAB Function/1(fh) -> Sum/1
  z3/1 -> Sum/2
  Sum/1 -> Gain1/1
  Gain1/1 -> Gain2/1
  Gain2/1 -> u/1

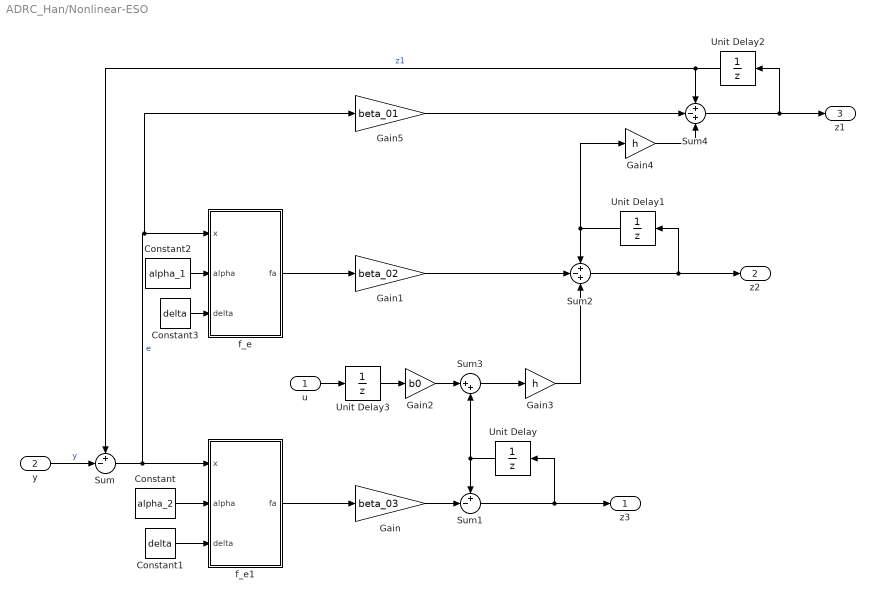
== system ADRC_Han/Nonlinear-ESO ==
  u : Inport
  y : Inport  Port=2
  Constant : Constant  Value=alpha_2
  Constant1 : Constant  Value=delta
  Constant2 : Constant  Value=alpha_1
  Constant3 : Constant  Value=delta
  Gain : Gain  Gain=beta_03
  Gain1 : Gain  Gain=beta_02
  Gain2 : Gain  Gain=b0
  Gain3 : Gain  Gain=h
  Gain4 : Gain  Gain=h
  Gain5 : Gain  Gain=beta_01
  Sum : Sum  Inputs=+-|
  Sum1 : Sum  Inputs=+-|
  Sum2 : Sum  Inputs=+-+
  Sum3 : Sum  Inputs=|++
  Sum4 : Sum  Inputs=+-+
  Unit Delay : UnitDelay  SampleTime=h  HasFrameUpgradeWarning=on
  Unit Delay1 : UnitDelay  SampleTime=-1  HasFrameUpgradeWarning=on
  Unit Delay2 : UnitDelay  SampleTime=-1  HasFrameUpgradeWarning=on
  Unit Delay3 : UnitDelay  SampleTime=-1  HasFrameUpgradeWarning=on
  f_e : MATLAB Function  TreatAsAtomicUnit=on
  f_e1 : MATLAB Function  TreatAsAtomicUnit=on
  z3 : Outport
  z2 : Outport  Port=2
  z1 : Outport  Port=3
  wires:
  Unit Delay2/1 -> Sum/1, Sum4/1  "z1"
  y/1 -> Sum/2  "y"
  Sum/1 -> Gain5/1, f_e/1(x), f_e1/1(x)  "e"
  Constant/1 -> f_e1/2(alpha)
  Constant1/1 -> f_e1/3(delta)
  f_e1/1(fa) -> Gain/1
  Gain/1 -> Sum1/2
  Sum1/1 -> z3/1, Unit Delay/1
  Unit Delay/1 -> Sum3/2, Sum1/1
  Constant2/1 -> f_e/2(alpha)
  Constant3/1 -> f_e/3(delta)
  f_e/1(fa) -> Gain1/1
  Gain1/1 -> Sum2/2
  u/1 -> Unit Delay3/1
  Gain2/1 -> Sum3/1
  Sum3/1 -> Gain3/1
  Gain3/1 -> Sum2/3
  Unit Delay1/1 -> Gain4/1, Sum2/1
  Sum2/1 -> z2/1, Unit Delay1/1
  Gain5/1 -> Sum4/2
  Gain4/1 -> Sum4/3
  Sum4/1 -> z1/1, Unit Delay2/1
  Unit Delay3/1 -> Gain2/1

== system ADRC_Han/TD ==
  ref : Inport
  Constant : Constant  Value=r0
  Constant1 : Constant  Value=h0
  Gain : Gain  Gain=h
  Gain1 : Gain  Gain=h
  MATLAB Function : MATLAB Function  TreatAsAtomicUnit=on  SystemSampleTime=h
  Sum : Sum  Inputs=+-|
  Sum1 : Sum  Inputs=++|
  Sum2 : Sum  Inputs=++|
  Unit Delay : UnitDelay  SampleTime=h  HasFrameUpgradeWarning=on
  Unit Delay1 : UnitDelay  SampleTime=h  HasFrameUpgradeWarning=on
  v1 : Outport
  v2 : Outport  Port=2
  wires:
  Sum/1 -> MATLAB Function/1(v1)
  ref/1 -> Sum/2
  Sum2/1 -> v1/1, Unit Delay/1  "v1(k)"
  MATLAB Function/1(fh) -> Gain/1
  Gain/1 -> Sum1/2
  Unit Delay1/1 -> Gain1/1, MATLAB Function/2(v2), Sum1/1  "v2(k-1)"
  Sum1/1 -> v2/1, Unit Delay1/1  "v2(k)"
  Gain1/1 -> Sum2/2
  Unit Delay/1 -> Sum/1, Sum2/1  "v1(k-1)"
  Constant/1 -> MATLAB Function/3(r0)
  Constant1/1 -> MATLAB Function/4(h0)

== matlab function ADRC_Han/NLSEF/MATLAB Function ==
  data: e1 input; e2 input; fh output; r input; h input
function fh = fhan(e1, e2, r, h)

d = h * r^2;
a0 = h * e2;
y = e1 + a0;

a1 = sqrt(d * (d + 8*abs(y)));
a2 = a0 + sign(y) * (a1 - d) / 2;
sy = (sign(y+d) - sign(y-d)) / 2;
a = (a0 + y - a2)*sy + a2;
sa = (sign(a+d) - sign(a-d)) / 2;
fh = -r * (a/d - sign(a)) * sa - r * sign(a);

== matlab function ADRC_Han/TD/MATLAB Function ==
  data: v1 input; v2 input; fh output; r0 input; h0 input
function fh = fhan(v1, v2, r0, h0)

d = h0 * r0^2;
a0 = h0 * v2;
y = v1 + a0;

a1 = sqrt(d * (d + 8*abs(y)));
a2 = a0 + sign(y) * (a1 - d) / 2;
sy = (sign(y+d) - sign(y-d)) / 2;
a = (a0 + y - a2)*sy + a2;
sa = (sign(a+d) - sign(a-d)) / 2;
fh = -r0 * (a/d - sign(a)) * sa - r0 * sign(a);

== matlab function ADRC_Han/Nonlinear-ESO/f_e1 ==
  data: x input; fa output; alpha input; delta input
function fa = fal(x, alpha, delta)

if abs(x) <= delta
    fa = x/(delta^(1-alpha));
else
    fa = abs(x)^alpha * sign(x);
end

== matlab function ADRC_Han/Nonlinear-ESO/f_e ==
  data: x input; fa output; alpha input; delta input
function fa = fal(x, alpha, delta)

if abs(x) <= delta
    fa = x/(delta^(1-alpha));
else
    fa = abs(x)^alpha * sign(x);
end
